simulink model "Conduction_Losses"  (R2015a)
settings: Solver=ode45  StartTime=0.0  StopTime=10.0  RelTol=1e-3
libraries: simulink x6
settings Model: Creator=Caner  LastModifiedBy=Caner

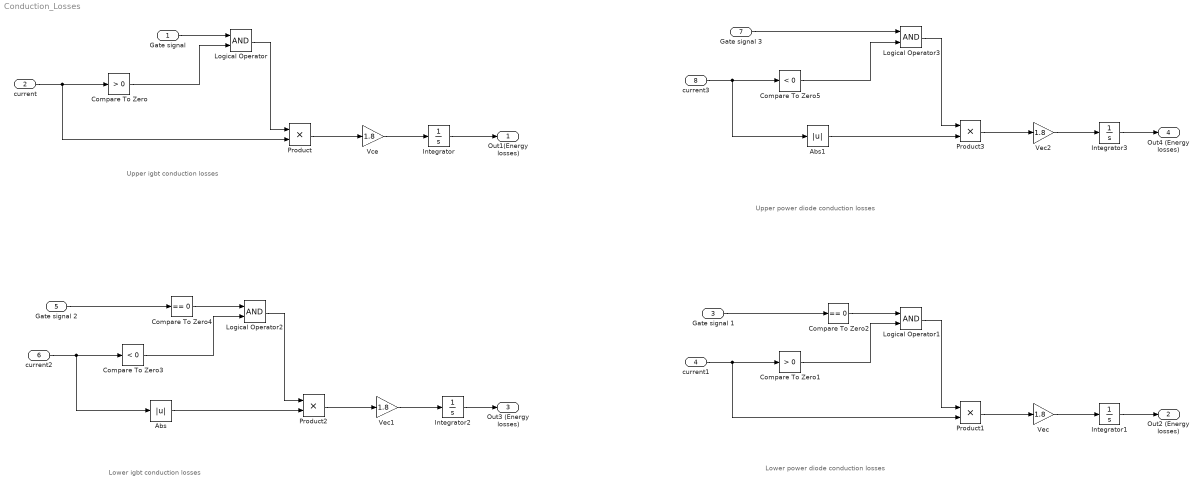
== system Conduction_Losses ==
  note: Upper power diode conduction losses
  note: Lower igbt conduction losses
  note: Lower power diode conduction losses
  note: Upper igbt conduction losses
  "Gate signal " : Inport
  current : Inport  Port=2
  Gate signal 1 : Inport  Port=3
  current1 : Inport  Port=4
  Gate signal 2 : Inport  Port=5
  current2 : Inport  Port=6
  Gate signal 3 : Inport  Port=7
  current3 : Inport  Port=8
  Abs : Abs
  Abs1 : Abs
  Compare To Zero : simulink/Logic and Bit Operations/Compare To Zero  relop=>  OutDataTypeStr=boolean
  Compare To Zero1 : simulink/Logic and Bit Operations/Compare To Zero  relop=>  OutDataTypeStr=boolean
  Compare To Zero2 : simulink/Logic and Bit Operations/Compare To Zero  relop===  OutDataTypeStr=boolean
  Compare To Zero3 : simulink/Logic and Bit Operations/Compare To Zero  relop=<  OutDataTypeStr=boolean
  Compare To Zero4 : simulink/Logic and Bit Operations/Compare To Zero  relop===  OutDataTypeStr=boolean
  Compare To Zero5 : simulink/Logic and Bit Operations/Compare To Zero  relop=<  OutDataTypeStr=boolean
  Integrator{,1..3} (4 alike) : Integrator
  Logical Operator{,1..3} (4 alike) : Logic  AllPortsSameDT=off  OutDataTypeStr=boolean
  Product{,1..3} (4 alike) : Product
  Vce : Gain  Gain=1.8
  Vec : Gain  Gain=1.8
  Vec1 : Gain  Gain=1.8
  Vec2 : Gain  Gain=1.8
  Out1(Energy losses) : Outport
  Out2 (Energy losses) : Outport  Port=2
  Out3 (Energy losses) : Outport  Port=3
  Out4 (Energy losses) : Outport  Port=4
  wires:
  current/1 -> Product/2, Compare To Zero/1
  "Gate signal "/1 -> Logical Operator/1
  Compare To Zero/1 -> Logical Operator/2
  Logical Operator/1 -> Product/1
  Product/1 -> Vce/1
  Vce/1 -> Integrator/1
  Integrator/1 -> Out1(Energy losses)/1
  current1/1 -> Product1/2, Compare To Zero1/1
  Gate signal 1/1 -> Compare To Zero2/1
  Compare To Zero1/1 -> Logical Operator1/2
  Logical Operator1/1 -> Product1/1
  Product1/1 -> Vec/1
  Vec/1 -> Integrator1/1
  Integrator1/1 -> Out2 (Energy losses)/1
  Compare To Zero2/1 -> Logical Operator1/1
  current2/1 -> Abs/1, Compare To Zero3/1
  Gate signal 2/1 -> Compare To Zero4/1
  Compare To Zero3/1 -> Logical Operator2/2
  Logical Operator2/1 -> Product2/1
  Product2/1 -> Vec1/1
  Vec1/1 -> Integrator2/1
  Integrator2/1 -> Out3 (Energy losses)/1
  Compare To Zero4/1 -> Logical Operator2/1
  Abs/1 -> Product2/2
  current3/1 -> Abs1/1, Compare To Zero5/1
  Compare To Zero5/1 -> Logical Operator3/2
  Logical Operator3/1 -> Product3/1
  Product3/1 -> Vec2/1
  Vec2/1 -> Integrator3/1
  Integrator3/1 -> Out4 (Energy losses)/1
  Abs1/1 -> Product3/2
  Gate signal 3/1 -> Logical Operator3/1
